simulink model "q_rotpen_swingup_student"  (Simulink 7.9)
settings: Solver=ode1  StartTime=0.0  StopTime=inf  FixedStep=0.002  RelTol=1e-3
PostLoadFcn:
  | qc_set_target_type(getConfigSet(bdroot, 'QUARC Default Target Configuration'));
undefined symbols (not defined in the file or in its folder): a_max, epsilon, Er, HIL, K, K_AMP, K_ENC, wcf_1, wcf_2
libraries: quarc_library x5, simulink_extras x3, simulink x3
settings Model: Creator=MLevis  LastModifiedBy=User  SimulationMode=external  ExtModeTrigDuration=10000
settings SolverCC: PositivePriorityOrder=on
settings OptimizationCC: InitFltsAndDblsToZero=on
settings DebuggingCC: SaveWithParameterizedLinksMsg=none  MultiTaskDSMMsg=warning  MultiTaskCondExecSysMsg=none  FcnCallInpInsideContextMsg=Use local settings  StrictBusMsg=None
settings RTWCC: SystemTargetFile=quarc_win64.tlc  TemplateMakefile=quarc_default_tmf  Description=QUARC Win64 Target  ProcessScript=quarc_win64_make_rtw_hook
settings STFCustomTargetCC: TargetPreCompLibLocation=C:\PROGRA~3\QUARC\lib\2012a\win64\release  CodeReplacementLibrary=ANSI_C  GeneratePreprocessorConditionals=Disable all  SystemTargetFile=quarc_win64.tlc
settings GRTTargetCC: TargetPreCompLibLocation=C:\PROGRA~3\QUARC\lib\2012a\win64\release  ParMdlRefBuildCompliant=off  CompOptLevelCompliant=off  ConcurrentExecutionCompliant=off  CombineOutputUpdateFcns=off  MatFileLogging=off  GRTInterface=on  ExtMode=on  ExtModeMexFile=quarc_comm

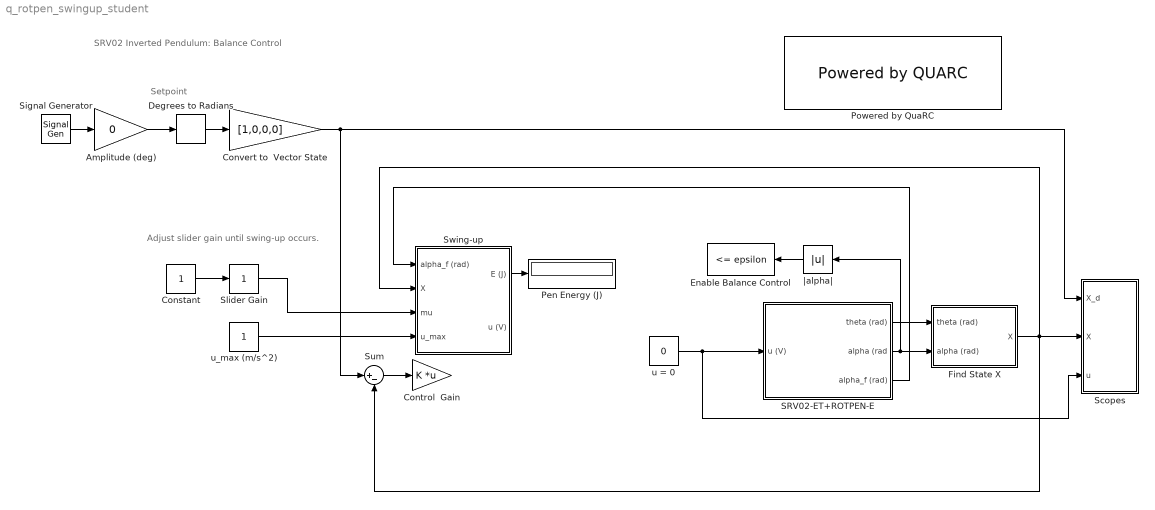
== system q_rotpen_swingup_student ==
  note: Setpoint
  note: SRV02 Inverted Pendulum: Balance Control
  note: Adjust slider gain
      | until swing-up occurs.
  Amplitude (deg) : Gain  Gain=0  SaturateOnIntegerOverflow=on  OutDataTypeStr=Inherit: Same as input  ParamDataTypeStr=Inherit: Same as input
  Constant : Constant
  Control  Gain : Gain  Gain=K  Multiplication=Matrix(K*u)
  Convert to  Vector State : Gain  Gain=[1,0,0,0]
  Degrees to Radians : simulink_extras/Transformations/Degrees to Radians
  Enable Balance Control : simulink/Logic and Bit Operations/Compare To Constant  relop=<=  const=epsilon  OutDataTypeStr=uint8  ZeroCross=off
  Find State X : Subsystem
  Pen Energy (J) : Display
      settings: Decimation=100
  Powered by QuaRC : quarc_library/Logos/Powered by QUARC
  SRV02-ET+ROTPEN-E : Subsystem
  Scopes : Subsystem
  Signal Generator : SignalGenerator  WaveForm=square  Frequency=0.1
  Slider Gain : simulink/Math Operations/Slider Gain  low=0  gain=1  high=10
  Sum : Sum  Inputs=|+-
  Swing-up : Subsystem
  u = 0 : Constant  Value=0
  u_max (m/s^2) : Constant
  |alpha| : Abs
  wires:
  Amplitude (deg)/1 -> Degrees to Radians/1
  Signal Generator/1 -> Amplitude (deg)/1
  Degrees to Radians/1 -> Convert to  Vector State/1
  Convert to  Vector State/1 -> Scopes/1(X_d), Sum/1
  Find State X/1(X) -> Scopes/2(X), Sum/2, Swing-up/2(X)
  SRV02-ET+ROTPEN-E/1(theta (rad)) -> Find State X/1(theta (rad))
  SRV02-ET+ROTPEN-E/2(alpha (rad) -> Find State X/2(alpha (rad)), |alpha|/1
  Sum/1 -> Control  Gain/1
  u = 0/1 -> Scopes/3(u), SRV02-ET+ROTPEN-E/1(u (V))
  |alpha|/1 -> Enable Balance Control/1
  SRV02-ET+ROTPEN-E/3(alpha_f (rad)) -> Swing-up/1(alpha_f (rad))
  Constant/1 -> Slider Gain/1
  Slider Gain/1 -> Swing-up/3(mu)
  Swing-up/1(E (J)) -> Pen Energy (J)/1
  u_max (m/s^2)/1 -> Swing-up/4(u_max)

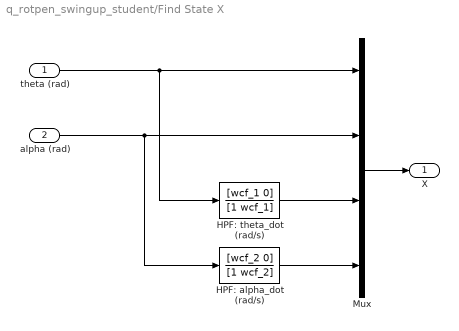
== system q_rotpen_swingup_student/Find State X ==
  theta (rad) : Inport
  alpha (rad) : Inport  Port=2
  HPF: alpha_dot (rad/s) : TransferFcn  Numerator=[wcf_2 0]  Denominator=[1 wcf_2]
  HPF: theta_dot (rad/s) : TransferFcn  Numerator=[wcf_1 0]  Denominator=[1 wcf_1]
  Mux : Mux
  X : Outport
  wires:
  alpha (rad)/1 -> Mux/2, HPF: alpha_dot (rad/s)/1
  Mux/1 -> X/1
  theta (rad)/1 -> Mux/1, HPF: theta_dot (rad/s)/1
  HPF: theta_dot (rad/s)/1 -> Mux/3
  HPF: alpha_dot (rad/s)/1 -> Mux/4

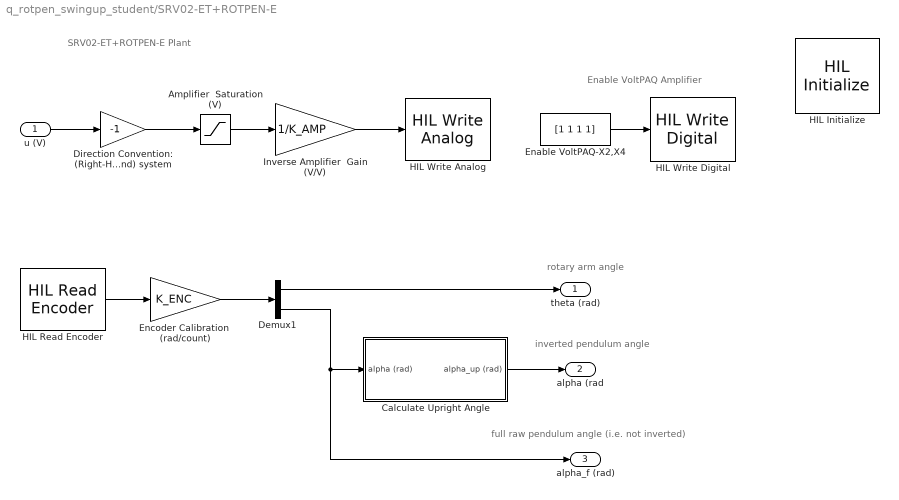
== system q_rotpen_swingup_student/SRV02-ET+ROTPEN-E ==
  note: SRV02-ET+ROTPEN-E Plant
  note: Enable VoltPAQ Amplifier
  note: inverted pendulum angle
  note: rotary arm angle
  note: full raw pendulum angle
      |  (i.e. not inverted)
  u (V) : Inport
  Amplifier  Saturation (V) : Saturate  UpperLimit=5  LowerLimit=-5
  Calculate Upright Angle : Subsystem
  Demux1 : Demux  Outputs=2
  Direction Convention: (Right-Hand) system : Gain  Gain=-1  SaturateOnIntegerOverflow=on  OutDataTypeStr=Inherit: Same as input  ParamDataTypeStr=Inherit: Same as input
  Enable VoltPAQ-X2,X4 : Constant  Value=[1 1 1 1]
  Encoder Calibration  (rad/count) : Gain  Gain=K_ENC  SaturateOnIntegerOverflow=on  OutDataTypeStr=Inherit: Same as input  ParamDataTypeStr=Inherit: Same as input
  HIL Initialize : quarc_library/Data Acquisition/Generic/Configuration/HIL Initialize  object_name=HIL-1  board_type=q8_usb  board_number=0  board_options=update_rate=normal  exclusive=off  active=off  hardware_clocks=[0:2]  clock_modes=[]  initial_clock_frequencies=[]  set_clock_params_at_start=off  set_clock_params_at_switch_in=off  set_clock_frequencies_at_start=off  set_clock_frequencies_at_switch_in=off  analog_input_channels=[0:7]  analog_input_maximums=10  analog_input_minimums=-10  set_analog_input_params_at_start=on  set_analog_input_params_at_switch_in=off  analog_output_channels=[0:7]  analog_output_maximums=10  analog_output_minimums=-10  initial_analog_outputs=[0]  final_analog_outputs=[0]  watchdog_analog_outputs=0  set_analog_output_params_at_start=on  set_analog_output_params_at_switch_in=off  set_analog_outputs_at_start=on  set_analog_outputs_at_switch_in=off  set_analog_outputs_at_terminate=on  set_analog_outputs_at_switch_out=off  set_analog_outputs_on_watchdog=off  digital_input_channels=[]  digital_output_channels=[0:7]  digital_output_configuration=[]  initial_digital_outputs=[0]  final_digital_outputs=[0]  watchdog_digital_outputs=[0]  set_digital_output_params_at_start=off  set_digital_output_params_at_switch_in=off  set_digital_outputs_at_start=on  set_digital_outputs_at_switch_in=off  set_digital_outputs_at_terminate=on  set_digital_outputs_at_switch_out=off  set_digital_outputs_on_watchdog=off  encoder_channels=[0:7]  quadrature=[4]  encoder_filter_frequency=[]  initial_encoder_counts=[0]  set_encoder_params_at_start=on  set_encoder_params_at_switch_in=off  set_encoder_counts_at_start=on  set_encoder_counts_at_switch_in=off  pwm_channels=[0:7]  pwm_modes=0  pwm_frequency=99.532799999999995e6/4095  pwm_configuration=[0]  pwm_alignment=[0]  pwm_polarity=[1]  pwm_leading_deadband=[0]  pwm_trailing_deadband=[0]  initial_pwm_outputs=[0]  final_pwm_outputs=[0]  watchdog_pwm_outputs=[0]  set_pwm_params_at_start=on  set_pwm_params_at_switch_in=off  set_pwm_outputs_at_start=on  set_pwm_outputs_at_switch_in=off  set_pwm_outputs_at_terminate=on  set_pwm_outputs_at_switch_out=off  set_pwm_outputs_on_watchdog=off  other_output_channels=[]  initial_other_outputs=[]  final_other_outputs=[]  watchdog_other_outputs=[]  set_other_outputs_at_start=off  set_other_outputs_at_switch_in=off  set_other_outputs_at_terminate=off  set_other_outputs_at_switch_out=off  set_other_outputs_on_watchdog=off
  HIL Read Encoder : quarc_library/Data Acquisition/Generic/Immediate I//O/HIL Read Encoder  object_name=HIL-1  channels=[0:1]  sample_time=qc_get_step_size  active=on  vector_output=on  data_type_mode=Inherit via back propagation  data_type=double
  HIL Write Analog : quarc_library/Data Acquisition/Generic/Immediate I//O/HIL Write Analog  object_name=HIL-1  channels=0  sample_time=-1  active=off  vector_input=off
  HIL Write Digital : quarc_library/Data Acquisition/Generic/Immediate I//O/HIL Write Digital  object_name=HIL-1  channels=[0:3]  sample_time=-1  active=off  vector_input=on
  Inverse Amplifier  Gain (V/V) : Gain  Gain=1/K_AMP
  theta (rad) : Outport
  alpha (rad : Outport  Port=2
  alpha_f (rad) : Outport  Port=3
  wires:
  Encoder Calibration  (rad/count)/1 -> Demux1/1
  Demux1/2 -> Calculate Upright Angle/1(alpha (rad)), alpha_f (rad)/1
  Enable VoltPAQ-X2,X4/1 -> HIL Write Digital/1
  HIL Read Encoder/1 -> Encoder Calibration  (rad/count)/1
  Amplifier  Saturation (V)/1 -> Inverse Amplifier  Gain (V/V)/1
  Inverse Amplifier  Gain (V/V)/1 -> HIL Write Analog/1
  u (V)/1 -> Direction Convention: (Right-Hand) system/1
  Direction Convention: (Right-Hand) system/1 -> Amplifier  Saturation (V)/1
  Demux1/1 -> theta (rad)/1
  Calculate Upright Angle/1(alpha_up (rad)) -> alpha (rad/1

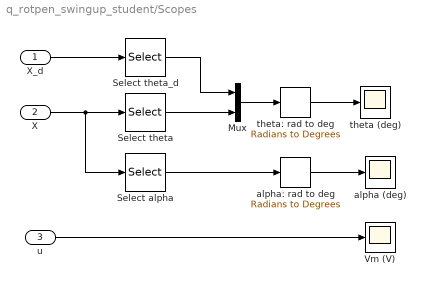
== system q_rotpen_swingup_student/Scopes ==
  X_d : Inport
  X : Inport  Port=2
  u : Inport  Port=3
  Mux : Mux  Inputs=2
  Select alpha : Selector  InputPortWidth=4  IndexOptions=Index vector (dialog)  Indices=2  OutputSizes=[(-2)]
  Select theta : Selector  InputPortWidth=4  IndexOptions=Index vector (dialog)  Indices=1  OutputSizes=[(-2)]
  Select theta_d : Selector  InputPortWidth=4  IndexOptions=Index vector (dialog)  Indices=1  OutputSizes=[(-2)]
  Vm (V) : Scope
      settings: TickLabels=on  TimeRange=10  SaveName=ScopeData3
  alpha (deg) : Scope
      settings: TimeRange=10  YMin=-200  YMax=200
  alpha: rad to deg : simulink_extras/Transformations/Radians to Degrees
  theta (deg) : Scope
      settings: YMin=-80  YMax=70
  theta: rad to deg : simulink_extras/Transformations/Radians to Degrees
  wires:
  u/1 -> Vm (V)/1
  X_d/1 -> Select theta_d/1
  Mux/1 -> theta: rad to deg/1
  Select alpha/1 -> alpha: rad to deg/1
  alpha: rad to deg/1 -> alpha (deg)/1
  X/1 -> Select alpha/1, Select theta/1
  Select theta_d/1 -> Mux/1
  theta: rad to deg/1 -> theta (deg)/1
  Select theta/1 -> Mux/2

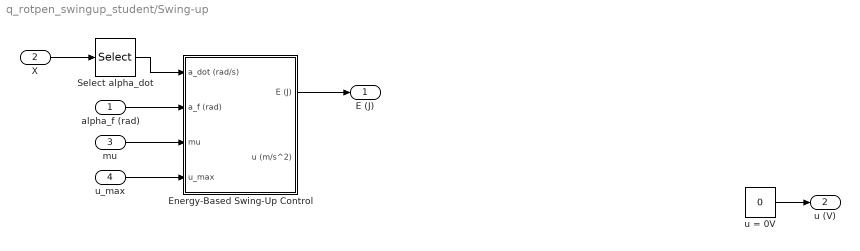
== system q_rotpen_swingup_student/Swing-up ==
  alpha_f (rad) : Inport
  X : Inport  Port=2
  mu : Inport  Port=3
  u_max : Inport  Port=4
  Energy-Based Swing-Up Control : Subsystem
  Select alpha_dot : Selector  InputPortWidth=4  IndexOptions=Index vector (dialog)  Indices=[4]  OutputSizes=1
  u = 0V : Constant  Value=0
  E (J) : Outport
  u (V) : Outport  Port=2
  wires:
  Energy-Based Swing-Up Control/1(E (J)) -> E (J)/1
  alpha_f (rad)/1 -> Energy-Based Swing-Up Control/2(a_f (rad))
  mu/1 -> Energy-Based Swing-Up Control/3(mu)
  Select alpha_dot/1 -> Energy-Based Swing-Up Control/1(a_dot (rad/s))
  X/1 -> Select alpha_dot/1
  u_max/1 -> Energy-Based Swing-Up Control/4(u_max)
  u = 0V/1 -> u (V)/1

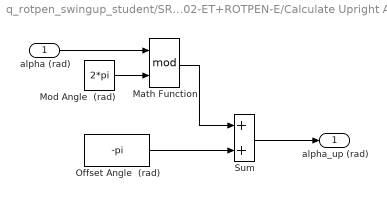
== system q_rotpen_swingup_student/SRV02-ET+ROTPEN-E/Calculate Upright Angle ==
  alpha (rad) : Inport
  Math Function : Math  Operator=mod  SaturateOnIntegerOverflow=on
  Mod Angle  (rad) : Constant  Value=2*pi
  Offset Angle  (rad) : Constant  Value=-pi
  Sum : Sum  SaturateOnIntegerOverflow=on  InputSameDT=on  OutDataTypeStr=Inherit: Same as first input
  alpha_up (rad) : Outport
  wires:
  Sum/1 -> alpha_up (rad)/1
  Mod Angle  (rad)/1 -> Math Function/2
  Offset Angle  (rad)/1 -> Sum/2
  alpha (rad)/1 -> Math Function/1
  Math Function/1 -> Sum/1

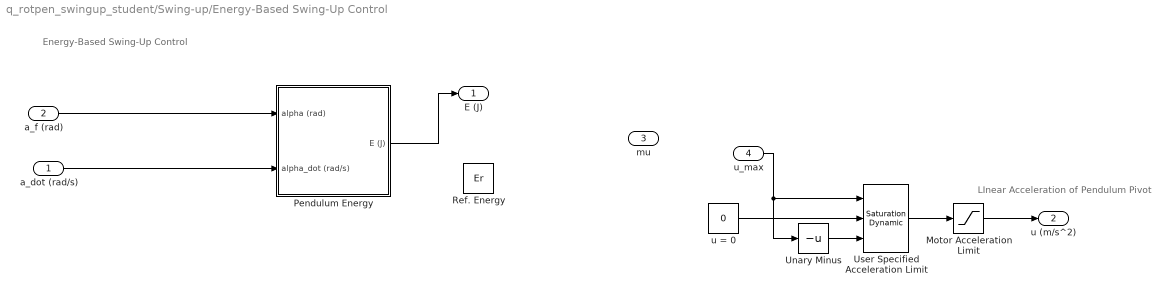
== system q_rotpen_swingup_student/Swing-up/Energy-Based Swing-Up Control ==
  note: Energy-Based Swing-Up Control
  note: LInear Acceleration of
      | Pendulum Pivot
  a_dot (rad/s) : Inport
  a_f (rad) : Inport  Port=2
  mu : Inport  Port=3
  u_max : Inport  Port=4
  Motor Acceleration Limit : Saturate  UpperLimit=a_max  LowerLimit=-a_max
  Pendulum Energy : Subsystem
  Ref. Energy : Constant  Value=Er
  Unary Minus : UnaryMinus
  User Specified Acceleration Limit : simulink/Discontinuities/Saturation Dynamic  OutMin=[]  OutMax=[]  OutDataTypeStr=Inherit: Same as second input  OutDataType=fixdt(1, 16)  OutScaling=2^-10  DoSatur=off
  u = 0 : Constant  Value=0
  E (J) : Outport
  u (m/s^2) : Outport  Port=2
  wires:
  a_f (rad)/1 -> Pendulum Energy/1(alpha (rad))
  Pendulum Energy/1(E (J)) -> E (J)/1
  a_dot (rad/s)/1 -> Pendulum Energy/2(alpha_dot (rad/s))
  u = 0/1 -> User Specified Acceleration Limit/2
  u_max/1 -> User Specified Acceleration Limit/1, Unary Minus/1
  Unary Minus/1 -> User Specified Acceleration Limit/3
  User Specified Acceleration Limit/1 -> Motor Acceleration Limit/1
  Motor Acceleration Limit/1 -> u (m/s^2)/1

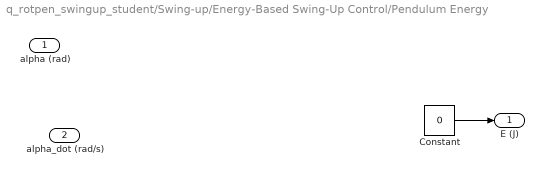
== system q_rotpen_swingup_student/Swing-up/Energy-Based Swing-Up Control/Pendulum Energy ==
  alpha (rad) : Inport
  alpha_dot (rad/s) : Inport  Port=2
  Constant : Constant  Value=0
  E (J) : Outport
  wires:
  Constant/1 -> E (J)/1
